simulink model "real_time_simulink"  (R2024b)
settings: Solver=ode5  StartTime=0.0  StopTime=7  FixedStep=0.001  RelTol=1e-3
values from neighbouring files (symbols this model uses):
  deltafil = 2^(-0.5)    (= 0.707106781187)    [LQR_code.m]    (also in PID_Luca.m)
  Kd = Kp * TD    [PID.m]
  Ki = Kp / TI    [PID.m]
  Kp = 1/(magP * magC)    [PID.m]
  Kw = 1/T_w    (= 7.14285714286)    [PID_Luca.m]
  omegac = 2*pi*50    (= 314.159265359)    [LQR_code.m]    (also in PID_Luca.m)
  t0 = 0.2    [Elastic_parameters_estimation.m]    (also in LQR_code.m; PID_Luca.m)
  t1 = 0.7    [Elastic_parameters_estimation.m]    (also in LQR_code.m; PID_Luca.m)
  tl = 1/(10*wgc)    [PID_Luca.m]
undefined symbols (not defined in the file or in its folder): degs2rpm, DiscIntNeverNeededParam, National_Instruments, PCI, pulse2deg, V2deg
libraries: sldrtlib x4, simulink x3
settings Model: SimulationMode=external  ExtModeTrigDuration=1000001  Creator=galeazzolu  LastModifiedBy=galeazzolu
settings DataIOCC: ReturnWorkspaceOutputs=off
settings HardwareCC: ProdBitPerLong=64  ProdHWDeviceType=Intel->x86-64 (Linux 64)
settings RTWCC: Description=Simulink Desktop Real-Time  SystemTargetFile=sldrt.tlc  TemplateMakefile=sldrt.tmf  RTWCompilerOptimization=on
settings CodeAppCC: MaxIdLength=95
settings SimulinkDesktopRealTimeCC: TargetLibSuffix=_sldrt.a  TargetPreCompLibLocation=C:\Program Files\MATLAB\R2024b\toolbox\sldrt\lib\win64  ParMdlRefBuildCompliant=on

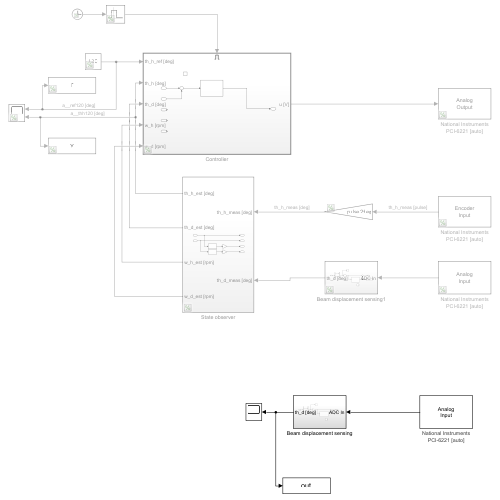
[thumbnail: Simulink's stored preview of the top-level diagram]
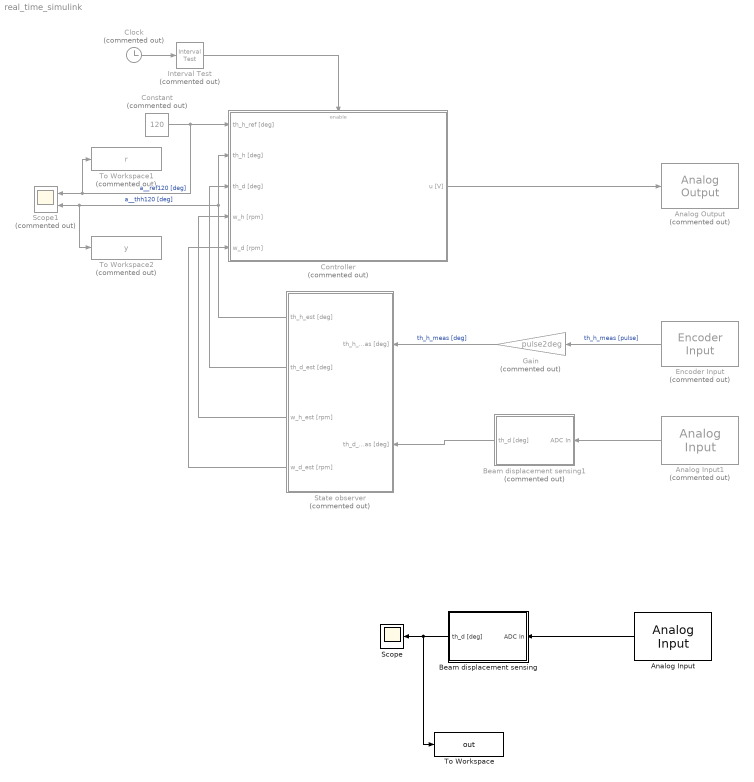
== system real_time_simulink ==
  Analog Input : sldrtlib/Analog Input  SampleTime=-1  MaxMissedTicks=10  ShowMissedTicks=off  YieldWhenWaiting=off  DrvName=National_Instruments/PCI-6221  DrvAddress=4294967295  DrvOptions=[0 0 0 2 0]  Channels=[3,4]  RangeMode=1  VoltRange=2  DataType=1
      settings: AttributesFormatString=National Instruments\nPCI-6221 [auto]
  Analog Input1 : sldrtlib/Analog Input  Commented=on  SampleTime=-1  MaxMissedTicks=10  ShowMissedTicks=off  YieldWhenWaiting=off  DrvName=National_Instruments/PCI-6221  DrvAddress=4294967295  DrvOptions=[0 0 0 2 0]  Channels=[3,4]  RangeMode=1  VoltRange=2  DataType=1
      settings: AttributesFormatString=National Instruments\nPCI-6221 [auto]
  Analog Output : sldrtlib/Analog Output  Commented=on  SampleTime=-1  MaxMissedTicks=10  ShowMissedTicks=off  YieldWhenWaiting=off  DrvName=National_Instruments/PCI-6221  DrvAddress=4294967295  DrvOptions=[0 0 0 2 0]  Channels=1  RangeMode=1  VoltRange=1  InitialValue=0  FinalValue=0
      settings: AttributesFormatString=National Instruments\nPCI-6221 [auto]
  Beam displacement sensing : Subsystem
  Beam displacement sensing1 : Subsystem  Commented=on
  Clock : Clock  Commented=on
  Constant : Constant  Commented=on  Value=120
  Controller : Subsystem  Commented=on  TreatAsAtomicUnit=on
  Encoder Input : sldrtlib/Encoder Input  Commented=on  SampleTime=-1  MaxMissedTicks=10  ShowMissedTicks=off  YieldWhenWaiting=off  DrvName=National_Instruments/PCI-6221  DrvAddress=4294967295  DrvOptions=[0 0 0 2 0]  Channels=1  QuadMode=3  IndexPulse=1  InputFilter=Inf  DataType=1
      settings: AttributesFormatString=National Instruments\nPCI-6221 [auto]
  Gain : Gain  Commented=on  Gain=pulse2deg
  Interval Test : simulink/Logic and Bit Operations/Interval Test  Commented=on  IntervalClosedRight=on  uplimit=inf  IntervalClosedLeft=on  lowlimit=t1  OutDataTypeStr=boolean
  Scope : Scope
  Scope1 : Scope  Commented=on  NumInputPorts=2
  State observer : Subsystem  Commented=on
  To Workspace : ToWorkspace  VariableName=out  SaveFormat=Structure With Time  SampleTime=-1
  To Workspace1 : ToWorkspace  Commented=on  VariableName=r  SaveFormat=Structure With Time  SampleTime=-1
  To Workspace2 : ToWorkspace  Commented=on  VariableName=y  SaveFormat=Structure With Time  SampleTime=-1
  wires:
  Beam displacement sensing1/1(th_d [deg]) -> State observer/2(th_d_meas [deg])
  Gain/1 -> State observer/1(th_h_meas [deg])  "th_h_meas [deg]"
  State observer/2(th_d_est [deg]) -> Controller/3(th_d [deg])
  State observer/1(th_h_est [deg]) -> Controller/2(th_h [deg]), To Workspace2/1, Scope1/2  "a__thh120 [deg]"
  Encoder Input/1 -> Gain/1  "th_h_meas [pulse]"
  State observer/4(w_d_est [rpm]) -> Controller/5(w_d [rpm])
  Analog Input/1 -> Beam displacement sensing/1(ADC In)
  State observer/3(w_h_est [rpm]) -> Controller/4(w_h [rpm])
  Clock/1 -> Interval Test/1
  Interval Test/1 -> Controller/Enable
  Constant/1 -> To Workspace1/1, Scope1/1, Controller/1(th_h_ref [deg])  "a__ref120 [deg]"
  Controller/1(u [V]) -> Analog Output/1
  Beam displacement sensing/1(th_d [deg]) -> To Workspace/1, Scope/1
  Analog Input1/1 -> Beam displacement sensing1/1(ADC In)

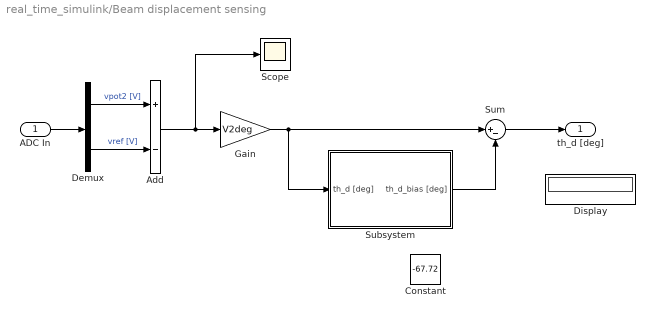
== system real_time_simulink/Beam displacement sensing ==
  ADC In : Inport
  Add : Sum  Inputs=+-
  Constant : Constant  Value=-67.72
  Demux : Demux  Outputs=2
  Display : Display
  Gain : Gain  Gain=V2deg
  Scope : Scope
  Subsystem : Subsystem
  Sum : Sum  Inputs=|+-
  th_d [deg] : Outport
  wires:
  ADC In/1 -> Demux/1
  Demux/1 -> Add/1  "vpot2 [V]"
  Demux/2 -> Add/2  "vref [V]"
  Add/1 -> Scope/1, Gain/1
  Gain/1 -> Subsystem/1(th_d [deg]), Sum/1
  Sum/1 -> th_d [deg]/1
  Subsystem/1(th_d_bias [deg]) -> Sum/2

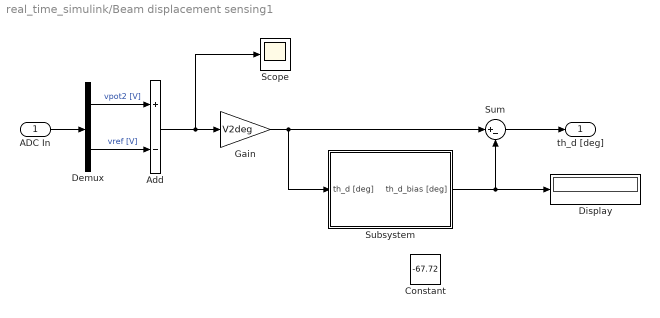
== system real_time_simulink/Beam displacement sensing1 ==
  ADC In : Inport
  Add : Sum  Inputs=+-
  Constant : Constant  Value=-67.72
  Demux : Demux  Outputs=2
  Display : Display
  Gain : Gain  Gain=V2deg
  Scope : Scope
  Subsystem : Subsystem
  Sum : Sum  Inputs=|+-
  th_d [deg] : Outport
  wires:
  Subsystem/1(th_d_bias [deg]) -> Sum/2, Display/1
  Sum/1 -> th_d [deg]/1
  Gain/1 -> Sum/1, Subsystem/1(th_d [deg])
  Add/1 -> Gain/1, Scope/1
  Demux/2 -> Add/2  "vref [V]"
  Demux/1 -> Add/1  "vpot2 [V]"
  ADC In/1 -> Demux/1

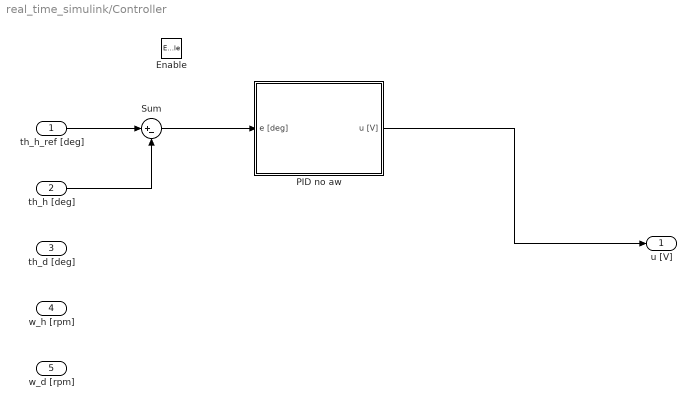
== system real_time_simulink/Controller ==
  th_h_ref [deg] : Inport
  th_h [deg] : Inport  Port=2
  th_d [deg] : Inport  Port=3
  w_h [rpm] : Inport  Port=4
  w_d [rpm] : Inport  Port=5
  Enable : EnablePort
  PID no aw : Subsystem
  Sum : Sum  Inputs=|+-
  u [V] : Outport
  wires:
  th_h_ref [deg]/1 -> Sum/1
  th_h [deg]/1 -> Sum/2
  Sum/1 -> PID no aw/1(e [deg])
  PID no aw/1(u [V]) -> u [V]/1

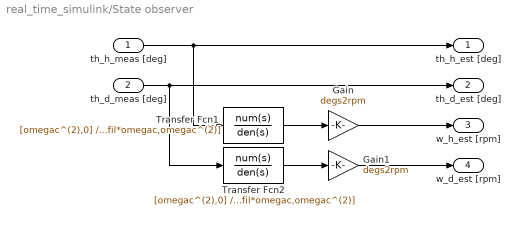
== system real_time_simulink/State observer ==
  th_h_meas [deg] : Inport
  th_d_meas [deg] : Inport  Port=2
  Gain : Gain  Gain=degs2rpm
  Gain1 : Gain  Gain=degs2rpm
  Transfer Fcn1 : TransferFcn  Numerator=[omegac^(2),0]  Denominator=[1,2*deltafil*omegac,omegac^(2)]
  Transfer Fcn2 : TransferFcn  Numerator=[omegac^(2),0]  Denominator=[1,2*deltafil*omegac,omegac^(2)]
  th_h_est [deg] : Outport
  th_d_est [deg] : Outport  Port=2
  w_h_est [rpm] : Outport  Port=3
  w_d_est [rpm] : Outport  Port=4
  wires:
  Transfer Fcn1/1 -> Gain/1
  Gain/1 -> w_h_est [rpm]/1
  Transfer Fcn2/1 -> Gain1/1
  Gain1/1 -> w_d_est [rpm]/1
  th_h_meas [deg]/1 -> Transfer Fcn1/1, th_h_est [deg]/1
  th_d_meas [deg]/1 -> Transfer Fcn2/1, th_d_est [deg]/1

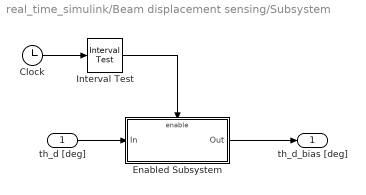
== system real_time_simulink/Beam displacement sensing/Subsystem ==
  th_d [deg] : Inport
  Clock : Clock
  Enabled Subsystem : Subsystem  TreatAsAtomicUnit=on
  Interval Test : simulink/Logic and Bit Operations/Interval Test  IntervalClosedRight=on  uplimit=t1  IntervalClosedLeft=on  lowlimit=t0  OutDataTypeStr=boolean
  th_d_bias [deg] : Outport
  wires:
  Interval Test/1 -> Enabled Subsystem/Enable
  Clock/1 -> Interval Test/1
  th_d [deg]/1 -> Enabled Subsystem/1(In)
  Enabled Subsystem/1(Out) -> th_d_bias [deg]/1

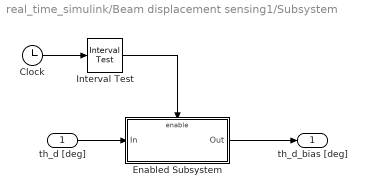
== system real_time_simulink/Beam displacement sensing1/Subsystem ==
  th_d [deg] : Inport
  Clock : Clock
  Enabled Subsystem : Subsystem  TreatAsAtomicUnit=on
  Interval Test : simulink/Logic and Bit Operations/Interval Test  IntervalClosedRight=on  uplimit=t1  IntervalClosedLeft=on  lowlimit=t0  OutDataTypeStr=boolean
  th_d_bias [deg] : Outport
  wires:
  Enabled Subsystem/1(Out) -> th_d_bias [deg]/1
  th_d [deg]/1 -> Enabled Subsystem/1(In)
  Clock/1 -> Interval Test/1
  Interval Test/1 -> Enabled Subsystem/Enable

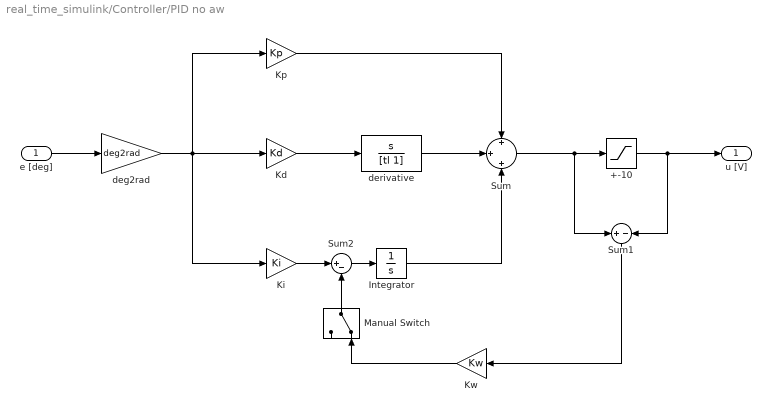
== system real_time_simulink/Controller/PID no aw ==
  e [deg] : Inport
  +-10 : Saturate  UpperLimit=10  LowerLimit=-10
  Integrator : Integrator
  Kd : Gain  Gain=Kd
  Ki : Gain  Gain=Ki
  Kp : Gain  Gain=Kp
  Kw : Gain  Gain=Kw
  Manual Switch : ManualSwitch  CurrentSetting=0
  Sum : Sum  Inputs=+|+|+
  Sum1 : Sum  Inputs=+|-
  Sum2 : Sum  Inputs=|+-
  deg2rad : Gain  Gain=deg2rad
  derivative : TransferFcn  Numerator=[1 0]  Denominator=[tl 1]
  u [V] : Outport
  wires:
  Kw/1 -> Manual Switch/2
  Integrator/1 -> Sum/3
  Sum2/1 -> Integrator/1
  e [deg]/1 -> deg2rad/1
  Kd/1 -> derivative/1
  Sum1/1 -> Kw/1
  Manual Switch/1 -> Sum2/2
  Sum/1 -> +-10/1, Sum1/1
  Ki/1 -> Sum2/1
  Kp/1 -> Sum/1
  deg2rad/1 -> Kd/1, Ki/1, Kp/1
  derivative/1 -> Sum/2
  +-10/1 -> Sum1/2, u [V]/1

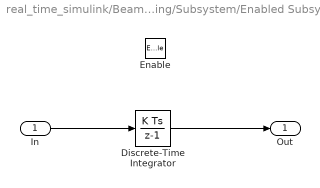
== system real_time_simulink/Beam displacement sensing/Subsystem/Enabled Subsystem ==
  In : Inport
  Enable : EnablePort
  Discrete-Time Integrator : DiscreteIntegrator  gainval=1/(t1-t0)  SampleTime=-1  ICPrevOutput=DiscIntNeverNeededParam  ICPrevScaledInput=DiscIntNeverNeededParam
  Out : Outport
  wires:
  In/1 -> Discrete-Time Integrator/1
  Discrete-Time Integrator/1 -> Out/1

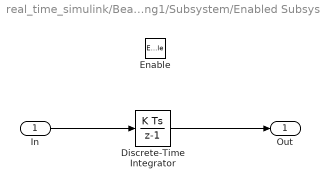
== system real_time_simulink/Beam displacement sensing1/Subsystem/Enabled Subsystem ==
  In : Inport
  Enable : EnablePort
  Discrete-Time Integrator : DiscreteIntegrator  gainval=1/(t1-t0)  SampleTime=-1  ICPrevOutput=DiscIntNeverNeededParam  ICPrevScaledInput=DiscIntNeverNeededParam
  Out : Outport
  wires:
  Discrete-Time Integrator/1 -> Out/1
  In/1 -> Discrete-Time Integrator/1
